simulink model "matlabarrayblock"  (R2022b)
settings: Solver=VariableStepAuto  StartTime=0.0  StopTime=10.0  RelTol=1e-3
settings Model: Creator=Brigosha_Guest  LastModifiedBy=Brigosha_Guest

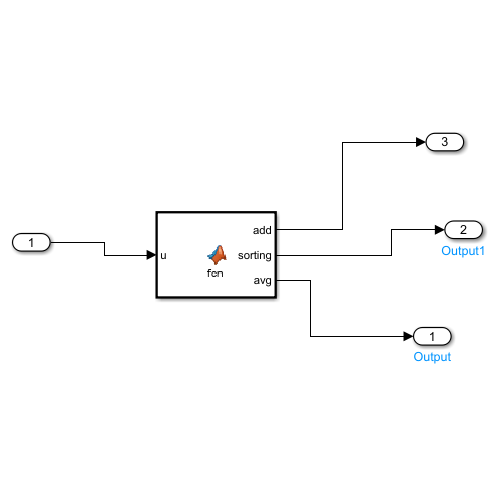
[thumbnail: Simulink's stored preview of the top-level diagram]
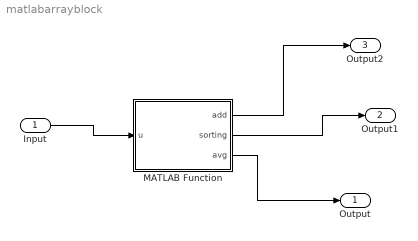
== system matlabarrayblock ==
  Input : Inport
  MATLAB Function : MATLAB Function  TreatAsAtomicUnit=on
  Output : Outport
  Output1 : Outport  Port=2
  Output2 : Outport  Port=3
  wires:
  Input/1 -> MATLAB Function/1(u)
  MATLAB Function/1(add) -> Output2/1
  MATLAB Function/2(sorting) -> Output1/1
  MATLAB Function/3(avg) -> Output/1

== matlab function matlabarrayblock/MATLAB Function ==
  data: u input; add output; sorting output; avg output
function [add,sorting,avg] = fcn(u)

add=sum(u);
sorting=sort(u);
avg=add/length(u);
